simulink model "ControlOblectSUBMod"  (R2023a)
settings: Solver=VariableStepAuto  StartTime=0.0  StopTime=10.0  RelTol=1e-3
settings Model: Creator=romav  LastModifiedBy=romav
settings DataIOCC: SaveOutput=off  SaveTime=off

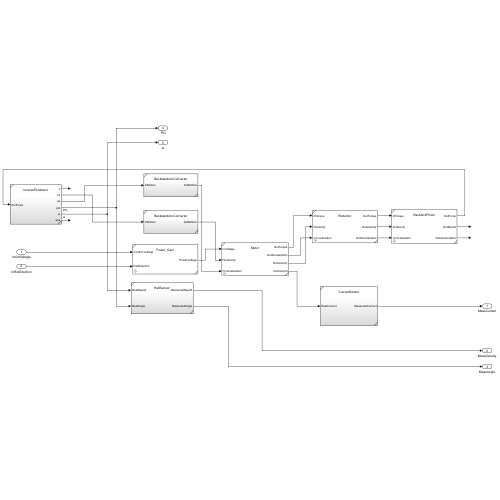
[thumbnail: Simulink's stored preview of the top-level diagram]
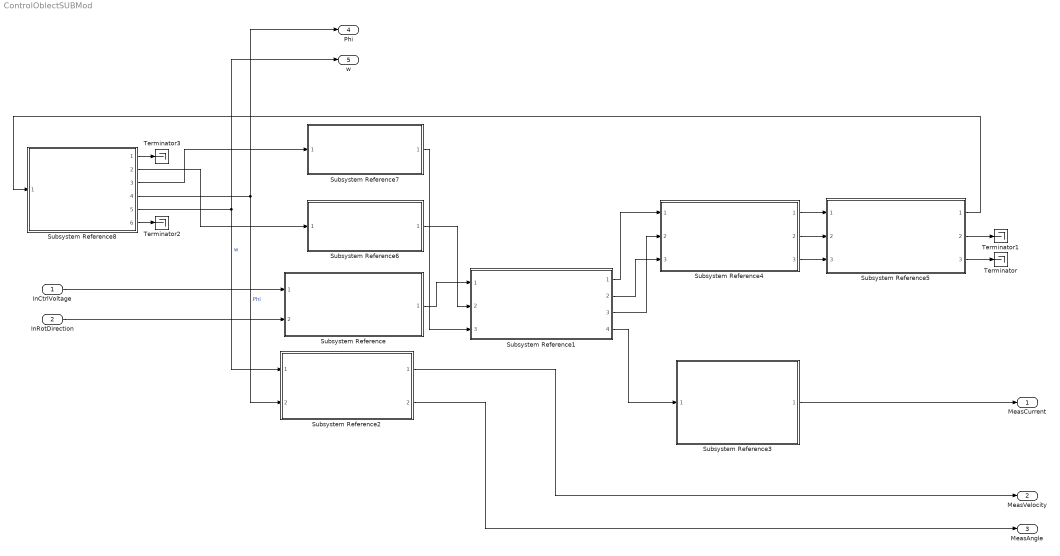
== system ControlOblectSUBMod ==
  InCtrlVoltage : Inport  OutDataTypeStr=double  PortDimensions=1  SampleTime=0
  InRotDirection : Inport  Port=2  OutDataTypeStr=double  PortDimensions=1  SampleTime=0
  Subsystem Reference : Subsystem  ReferencedSubsystem=Power_Gain  Kpa=7.3
  Subsystem Reference1 : Subsystem  ReferencedSubsystem=Motor  kw=62.8  km=16e-3  motor_nominal_voltage=24  vis_friction_coef_motor=0.1
  Subsystem Reference2 : Subsystem  ReferencedSubsystem=HallSensor
  Subsystem Reference3 : Subsystem  ReferencedSubsystem=CurrentSensor
  Subsystem Reference4 : Subsystem  ReferencedSubsystem=Reductor  i_gear=100  J_gear=2.4e-6  vis_friction_coef_gear=0.15
  Subsystem Reference5 : Subsystem  ReferencedSubsystem=RackAndPinion  i_rp=20000  vis_friction_coef_rp=0.002  J_pinion=1e-6
  Subsystem Reference6 : Subsystem  ReferencedSubsystem=BackwardAccConverter
  Subsystem Reference7 : Subsystem  ReferencedSubsystem=BackwardAccConverter
  Subsystem Reference8 : Subsystem  ReferencedSubsystem=InversePendulum
  Terminator{,1..3} (4 alike) : Terminator
  MeasCurrent : Outport  OutDataTypeStr=double  PortDimensions=1  SampleTime=0
  MeasVelocity : Outport  Port=2  OutDataTypeStr=double  PortDimensions=1  SampleTime=0
  MeasAngle : Outport  Port=3  OutDataTypeStr=double  PortDimensions=1  SampleTime=0
  " Phi" : Outport  Port=4  OutDataTypeStr=double  PortDimensions=1  SampleTime=0
  w : Outport  Port=5  OutDataTypeStr=double  PortDimensions=1  SampleTime=0
  wires:
  Subsystem Reference8/3 -> Subsystem Reference7/1
  Subsystem Reference1/4 -> Subsystem Reference3/1
  Subsystem Reference8/5 -> Subsystem Reference2/1, w/1  "w"
  Subsystem Reference8/6 -> Terminator2/1
  Subsystem Reference5/1 -> Subsystem Reference8/1
  Subsystem Reference6/1 -> Subsystem Reference1/2
  Subsystem Reference8/2 -> Subsystem Reference6/1
  Subsystem Reference/1 -> Subsystem Reference1/1
  Subsystem Reference8/4 -> Subsystem Reference2/2, " Phi"/1  "Phi"
  Subsystem Reference4/2 -> Subsystem Reference5/2
  Subsystem Reference4/3 -> Subsystem Reference5/3
  Subsystem Reference7/1 -> Subsystem Reference1/3
  Subsystem Reference3/1 -> MeasCurrent/1
  Subsystem Reference4/1 -> Subsystem Reference5/1
  Subsystem Reference1/3 -> Subsystem Reference4/2
  Subsystem Reference2/2 -> MeasAngle/1
  Subsystem Reference5/3 -> Terminator/1
  Subsystem Reference1/2 -> Subsystem Reference4/3
  Subsystem Reference5/2 -> Terminator1/1
  Subsystem Reference2/1 -> MeasVelocity/1
  Subsystem Reference1/1 -> Subsystem Reference4/1
  InRotDirection/1 -> Subsystem Reference/2
  InCtrlVoltage/1 -> Subsystem Reference/1
  Subsystem Reference8/1 -> Terminator3/1
